simulink model "PubIfDecisionTOS_MDL"  (R2020b)
settings: configuration reference "DspaceConfig" (kept outside this file)
PostLoadFcn:
  | if any(exist('dsrtsu_mdlpostloadfcn', 'file') ~= 0), dsrtsu_mdlpostloadfcn('Execute', bdroot); end
InitFcn:
  | , if any(exist('dsmpb_private', 'file') ~= 0), dsmpb_private('dsmpb_mdlclblib', 'Init', bdroot); end,
undefined symbols (not defined in the file or in its folder): C_TOS_ACCEgoRAxletoFbumplength_m, C_TOS_ACCTargetFront_Flag, C_TOS_AEBJAPedObjDxThre_Val, C_TOS_AEBJAPedObjDyThre_Val, C_TOS_AEBJATargetSize_Val, C_TOS_AEBJAVehObjDxThre_Val, C_TOS_AEBJAVehObjDyThre_Val, C_TOS_AEBJuncPedTargetSize_Val, C_TOS_AEBLatObjDxThre_Val, C_TOS_AEBLatPedDyThre_Val, C_TOS_AEBLatTargetSize_Val, C_TOS_AEBLongTargetInEgoFront_Flag, C_TOS_axAbsGround_Parameter, C_TOS_CameraConfirmedFlag, C_TOS_CNsubjWidth, C_TOS_CurrentLaneCoreMinWidth_Val, C_TOS_CutInProb_Val_Zero, C_TOS_CutOutProb_Val_Zero, C_TOS_D2R_Val, C_TOS_DefaultValueObjectToCenterLine_dy, C_TOS_EgoCarWidth_Val, C_TOS_EgoDxRefPoint_m, C_TOS_EgoRAxletoFbumplength_m, C_TOS_HalfWidthVehicle_Con, C_TOS_HWA_CurrentLaneFlag, C_TOS_HWA_LeftLaneFlag, C_TOS_HWA_MovingDir_Vaild, C_TOS_HWA_MovState_Vaild, C_TOS_HWA_RightLaneFlag, C_TOS_LaneLineCourseErrorFront, C_TOS_LaneLineCourseErrorRear, C_TOS_MotorbikeDefaultWidth_m, C_TOS_NumberOfEffectiveTargets, C_TOS_Obj_Age_Val, C_TOS_Objdx_Constraint_Val, C_TOS_ObjectDefaultWidth_m, C_TOS_ObjInCurrentLane_Val, C_TOS_ObjInCurrentLaneValid, C_TOS_ObjInLeftLaneValid, C_TOS_ObjInRightLaneValid, C_TOS_ObjNotInCurrentLane_Val, C_TOS_ObjNotREElementType, C_TOS_ObjPredictDis_dy_ConstantVal_Zeros, C_TOS_ObjToCenterLine_ConstantVal_Zeros, C_TOS_OFMObjIDInvilad_Val, C_TOS_PIL_LatDisCons_Val_zero, C_TOS_PIL_ObjectCutInFlag_b, C_TOS_PIL_ObjectCutOutFlag_b, C_TOS_PIL_ObjLaneProb_al_Val, C_TOS_PP_ObjFusType_FC_Confirm_b, C_TOS_PP_ObjFusType_FC_FR_Confirm_b, C_TOS_PP_ObjFusType_FR_Confirm_b, C_TOS_RE_80BoolDefault_Val, C_TOS_RE_80Single181Default_Val, C_TOS_RE_80Single255Default_Val, C_TOS_RE_80Uint8Default_Val, C_TOS_RE_D2R, C_TOS_RE_D_180_Val, C_TOS_RE_InvalidObjectID_Val, C_TOS_RE_InvalidTargetChainDir_Val ... (+142)
libraries: simulink x1650, TOS_LIB x361, canfdmsglib x14
(part 52 of 69)

== system PubIfDecisionTOS_MDL/TOS_20201112/TOS_2012080320/TOS/ACC/TOS_ACCRightLane/ACC_LeftLane_Target/TOS_ACC_P3/ACC_P3_Targe/ACC_P3_Targe/TOS_ACC_ObjTypeConfirm/Subsystem1 ==
  note: 针对有选中的运动目标，运动状态突变为静止，改变其运动状态为运动
  object_MovingState : Inport
  ACC_Target_ID_K1 : Inport  Port=2
  ACC_Target_ID_K2 : Inport  Port=3
  ACC_Target_MovState_K1 : Inport  Port=4
  ACC_Target_MovState_K2 : Inport  Port=5
  ObjectID : Inport  Port=6
  Object_Type : Inport  Port=7
  Compare To Constant11 : simulink/Logic and Bit Operations/Compare To Constant  relop===  const=1  OutDataTypeStr=boolean
  Compare To Constant2 : simulink/Logic and Bit Operations/Compare To Constant  relop===  const=OFM_OBJ_MOVINGSTATE_E.MOVING  OutDataTypeStr=boolean
      settings: AttributesFormatString=OFM_OBJ_MOVINGSTATE_E.MOVING = 2
  Compare To Constant3 : simulink/Logic and Bit Operations/Compare To Constant  relop===  const=OFM_OBJ_MOVINGSTATE_E.MOVING_SLOWLY  OutDataTypeStr=boolean
      settings: AttributesFormatString=OFM_OBJ_MOVINGSTATE_E.MOVING_SLOWLY = 5
  Compare To Constant6 : simulink/Logic and Bit Operations/Compare To Constant  relop===  const=OFM_OBJ_MOVINGSTATE_E.STOPPED  OutDataTypeStr=boolean
      settings: AttributesFormatString=OFM_OBJ_MOVINGSTATE_E.STOPPED = 4
  Compare To Constant8 : simulink/Logic and Bit Operations/Compare To Constant  relop===  const=OFM_OBJ_TYPE_E.UNKNOWN_TYPE  OutDataTypeStr=boolean
      settings: AttributesFormatString=OFM_OBJ_TYPE_E.UNKNOWN_TYPE = 1
  Data Type Conversion2 : DataTypeConversion  OutDataTypeStr=Enum: OFM_OBJ_MOVINGSTATE_E
  Logical Operator : Logic  AllPortsSameDT=off  OutDataTypeStr=boolean
  Logical Operator2 : Logic  Operator=OR  Inputs=4  AllPortsSameDT=off  OutDataTypeStr=boolean
  Subsystem : Subsystem
  Output : Outport
  wires:
  ACC_Target_MovState_K2/1 -> Subsystem/5(ACC_Target_MovState_K2)
  Subsystem/1(TOS_ObjMovStateCfm) -> Compare To Constant11/1
  Data Type Conversion2/1 -> Compare To Constant2/1, Compare To Constant3/1, Compare To Constant6/1, Subsystem/1(ObjMovState)
  ObjectID/1 -> [ObjectID], Subsystem/6(ObjectID)
  ACC_Target_ID_K1/1 -> Subsystem/2(ACC_Target_ID_K1), [ACC_Target_ID_K1]
  Compare To Constant11/1 -> Logical Operator2/4
  Logical Operator2/1 -> Logical Operator/1
  ACC_Target_MovState_K1/1 -> Subsystem/4(ACC_Target_MovState_K1)
  Compare To Constant2/1 -> Logical Operator2/1
  Compare To Constant3/1 -> Logical Operator2/2
  Compare To Constant8/1 -> Logical Operator/2
  ACC_Target_ID_K2/1 -> Subsystem/3(ACC_Target_ID_K2)
  object_MovingState/1 -> Data Type Conversion2/1
  Compare To Constant6/1 -> Logical Operator2/3
  Object_Type/1 -> Compare To Constant8/1
  Logical Operator/1 -> Output/1

== system PubIfDecisionTOS_MDL/TOS_20201112/TOS_2012080320/TOS/ACC/TOS_ACCRightLane/ACC_LeftLane_Target/TOS_ACC_P3/ACC_P3_Targe/ACC_P3_Targe/TOS_ACC_ObjTypeConfirm/TOS_ACCObjTypeAborDly ==
  ACC_Target_ID_K1 : Inport
  ObjectID : Inport  Port=2
  TOS_ACCObjType : Inport  Port=3
  If : If  IfExpression=u1
  If Action Subsystem : Subsystem  TreatAsAtomicUnit=on
  If Action Subsystem1 : Subsystem  TreatAsAtomicUnit=on
  Merge : Merge
  Relational Operator : RelationalOperator  Operator===  OutDataTypeStr=boolean  RndMeth=Simplest
  TOS_ACCObjTypeFilt : Outport
  wires:
  Merge/1 -> TOS_ACCObjTypeFilt/1
  If Action Subsystem/1(TOS_ACCFusionTypeFilt) -> Merge/2
  If Action Subsystem1/1(TOS_ACCFusionTypeFilt) -> Merge/1
  Relational Operator/1 -> If/1
  ObjectID/1 -> Relational Operator/2
  ACC_Target_ID_K1/1 -> Relational Operator/1
  If/2 -> If Action Subsystem/Action
  TOS_ACCObjType/1 -> If Action Subsystem/1(TOS_ACCFusionType), If Action Subsystem1/1(TOS_ACCFusionType)
  If/1 -> If Action Subsystem1/Action

== system PubIfDecisionTOS_MDL/TOS_20201112/TOS_2012080320/TOS/ACC/TOS_ACCRightLane/ACC_LeftLane_Target/TOS_ACC_P3/ACC_P3_Targe/ACC_P3_Targe/TOS_ACC_ObstacleProbConfirm/TOS_ACCObstacleProbAborDly ==
  ACC_Target_ID_K1 : Inport
  ObjectID : Inport  Port=2
  TOS_ACCObstacleProb : Inport  Port=3
  If : If  IfExpression=u1
  If Action Subsystem : Subsystem  TreatAsAtomicUnit=on
  If Action Subsystem1 : Subsystem  TreatAsAtomicUnit=on
  Merge : Merge
  Subsystem : Subsystem
  TOS_ACCObstacleProbFilt : Outport
  wires:
  Merge/1 -> TOS_ACCObstacleProbFilt/1
  If Action Subsystem/1(TOS_ACCFusionTypeFilt) -> Merge/2
  If Action Subsystem1/1(TOS_ACCFusionTypeFilt) -> Merge/1
  Subsystem/1(ACC_SameTargetP0) -> If/1
  ObjectID/1 -> Subsystem/2(ObjectID)
  ACC_Target_ID_K1/1 -> Subsystem/1(ACC_TargetP0_ID_K1)
  If/2 -> If Action Subsystem/Action
  TOS_ACCObstacleProb/1 -> If Action Subsystem/1(TOS_ACCFusionType), If Action Subsystem1/1(TOS_ACCFusionType)
  If/1 -> If Action Subsystem1/Action

== system PubIfDecisionTOS_MDL/TOS_20201112/TOS_2012080320/TOS/ACC/TOS_ACCRightLane/ACC_LeftLane_Target/TOS_ACC_P3/ACC_P3_Targe/ACC_P3_Targe/TOS_ACC_TargetMovingDirConfirm/Subsystem ==
  ObjMovState : Inport
  ACC_Target_ID_K1 : Inport  Port=2
  ACC_Target_ID_K2 : Inport  Port=3
  ACC_Target_MovState_K1 : Inport  Port=4
  ACC_Target_MovState_K2 : Inport  Port=5
  ObjectID : Inport  Port=6
  TOS_ObjMovStateCfmFlow : Stateflow chart  TreatAsAtomicUnit=on
  TOS_ObjMovStateCfm : Outport
  wires:
  ObjectID/1 -> TOS_ObjMovStateCfmFlow/6(ObjectID)
  ObjMovState/1 -> TOS_ObjMovStateCfmFlow/5(ObjMovState)
  ACC_Target_MovState_K2/1 -> TOS_ObjMovStateCfmFlow/4(Target_MovState_K2)
  ACC_Target_MovState_K1/1 -> TOS_ObjMovStateCfmFlow/3(Target_MovState_K1)
  ACC_Target_ID_K2/1 -> TOS_ObjMovStateCfmFlow/2(Target_ID_K2)
  ACC_Target_ID_K1/1 -> TOS_ObjMovStateCfmFlow/1(Target_ID_K1)
  TOS_ObjMovStateCfmFlow/1(TOS_ObjMovStateCfm) -> TOS_ObjMovStateCfm/1

== system PubIfDecisionTOS_MDL/TOS_20201112/TOS_2012080320/TOS/ACC/TOS_ACCRightLane/ACC_LeftLane_Target/TOS_ACC_P3/ACC_P3_Targe/ACC_P3_Targe/TOS_ACC_TargetMovingDirConfirm/TOS_ACCMovingDirAborDly ==
  ACC_TargetP0_ID_K1 : Inport
  ObjectID : Inport  Port=2
  TOS_ACCMovingDir : Inport  Port=3
  If : If  IfExpression=u1
  If Action Subsystem : Subsystem  TreatAsAtomicUnit=on
  If Action Subsystem1 : Subsystem  TreatAsAtomicUnit=on
  Merge : Merge
  Subsystem : Subsystem
  TOS_ACC_TrgMovDirFlag_6_ObserVale : Outport
  TOS_ACC_TrgMovDir : Outport  Port=2
  wires:
  Merge/1 -> TOS_ACC_TrgMovDir/1
  If Action Subsystem/1(TOS_ACCMovingDirFilt) -> Merge/2
  If Action Subsystem1/1(TOS_ACCMovingDirFilt) -> Merge/1
  Subsystem/1(ACC_SameTargetP0) -> If/1, TOS_ACC_TrgMovDirFlag_6_ObserVale/1
  ObjectID/1 -> Subsystem/2(ObjectID)
  ACC_TargetP0_ID_K1/1 -> Subsystem/1(ACC_TargetP0_ID_K1)
  If/2 -> If Action Subsystem/Action
  TOS_ACCMovingDir/1 -> If Action Subsystem/1(TOS_ACCMovingDir), If Action Subsystem1/1(TOS_ACCMovingDir)
  If/1 -> If Action Subsystem1/Action

== system PubIfDecisionTOS_MDL/TOS_20201112/TOS_2012080320/TOS/ACC/TOS_ACCRightLane/ACC_LeftLane_Target/TOS_ACC_P5/ACC_P5_Targe/ACC_P5_Targe/TOS_ACC_FusionTypeConfirm/Subsystem1 ==
  ObjMovState : Inport
  ACC_Target_ID_K1 : Inport  Port=2
  ACC_Target_ID_K2 : Inport  Port=3
  ACC_Target_MovState_K1 : Inport  Port=4
  ACC_Target_MovState_K2 : Inport  Port=5
  ObjectID : Inport  Port=6
  TOS_ObjMovStateCfmFlow1 : Stateflow chart  TreatAsAtomicUnit=on
  TOS_ObjMovStateCfm : Outport
  wires:
  TOS_ObjMovStateCfmFlow1/1(TOS_ObjMovStateCfm) -> TOS_ObjMovStateCfm/1
  ACC_Target_ID_K1/1 -> TOS_ObjMovStateCfmFlow1/1(Target_ID_K1)
  ACC_Target_ID_K2/1 -> TOS_ObjMovStateCfmFlow1/2(Target_ID_K2)
  ACC_Target_MovState_K1/1 -> TOS_ObjMovStateCfmFlow1/3(Target_MovState_K1)
  ACC_Target_MovState_K2/1 -> TOS_ObjMovStateCfmFlow1/4(Target_MovState_K2)
  ObjMovState/1 -> TOS_ObjMovStateCfmFlow1/5(ObjMovState)
  ObjectID/1 -> TOS_ObjMovStateCfmFlow1/6(ObjectID)

== system PubIfDecisionTOS_MDL/TOS_20201112/TOS_2012080320/TOS/ACC/TOS_ACCRightLane/ACC_LeftLane_Target/TOS_ACC_P5/ACC_P5_Targe/ACC_P5_Targe/TOS_ACC_FusionTypeConfirm/TOS_ACCFusionTypeAborDly ==
  ACC_TargetP0_ID_K1 : Inport
  ObjectID : Inport  Port=2
  TOS_ACCFusionType : Inport  Port=3
  If : If  IfExpression=u1
  If Action Subsystem : Subsystem  TreatAsAtomicUnit=on
  If Action Subsystem1 : Subsystem  TreatAsAtomicUnit=on
  Merge : Merge
  Relational Operator : RelationalOperator  Operator===  OutDataTypeStr=boolean  RndMeth=Simplest
  TOS_ACCFusionTypeFilt : Outport
  wires:
  If/1 -> If Action Subsystem1/Action
  TOS_ACCFusionType/1 -> If Action Subsystem1/1(TOS_ACCFusionType), If Action Subsystem/1(TOS_ACCFusionType)
  If/2 -> If Action Subsystem/Action
  ACC_TargetP0_ID_K1/1 -> Relational Operator/1
  ObjectID/1 -> Relational Operator/2
  Relational Operator/1 -> If/1
  If Action Subsystem1/1(TOS_ACCFusionTypeFilt) -> Merge/1
  If Action Subsystem/1(TOS_ACCFusionTypeFilt) -> Merge/2
  Merge/1 -> TOS_ACCFusionTypeFilt/1

== system PubIfDecisionTOS_MDL/TOS_20201112/TOS_2012080320/TOS/ACC/TOS_ACCRightLane/ACC_LeftLane_Target/TOS_ACC_P5/ACC_P5_Targe/ACC_P5_Targe/TOS_ACC_ObjTypeConfirm/Subsystem1 ==
  note: 针对有选中的运动目标，运动状态突变为静止，改变其运动状态为运动
  object_MovingState : Inport
  ACC_Target_ID_K1 : Inport  Port=2
  ACC_Target_ID_K2 : Inport  Port=3
  ACC_Target_MovState_K1 : Inport  Port=4
  ACC_Target_MovState_K2 : Inport  Port=5
  ObjectID : Inport  Port=6
  Object_Type : Inport  Port=7
  Compare To Constant11 : simulink/Logic and Bit Operations/Compare To Constant  relop===  const=1  OutDataTypeStr=boolean
  Compare To Constant2 : simulink/Logic and Bit Operations/Compare To Constant  relop===  const=OFM_OBJ_MOVINGSTATE_E.MOVING  OutDataTypeStr=boolean
      settings: AttributesFormatString=OFM_OBJ_MOVINGSTATE_E.MOVING = 2
  Compare To Constant3 : simulink/Logic and Bit Operations/Compare To Constant  relop===  const=OFM_OBJ_MOVINGSTATE_E.MOVING_SLOWLY  OutDataTypeStr=boolean
      settings: AttributesFormatString=OFM_OBJ_MOVINGSTATE_E.MOVING_SLOWLY = 5
  Compare To Constant6 : simulink/Logic and Bit Operations/Compare To Constant  relop===  const=OFM_OBJ_MOVINGSTATE_E.STOPPED  OutDataTypeStr=boolean
      settings: AttributesFormatString=OFM_OBJ_MOVINGSTATE_E.STOPPED = 4
  Compare To Constant8 : simulink/Logic and Bit Operations/Compare To Constant  relop===  const=OFM_OBJ_TYPE_E.UNKNOWN_TYPE  OutDataTypeStr=boolean
      settings: AttributesFormatString=OFM_OBJ_TYPE_E.UNKNOWN_TYPE = 1
  Data Type Conversion2 : DataTypeConversion  OutDataTypeStr=Enum: OFM_OBJ_MOVINGSTATE_E
  Logical Operator : Logic  AllPortsSameDT=off  OutDataTypeStr=boolean
  Logical Operator2 : Logic  Operator=OR  Inputs=4  AllPortsSameDT=off  OutDataTypeStr=boolean
  Subsystem : Subsystem
  Output : Outport
  wires:
  Logical Operator/1 -> Output/1
  Object_Type/1 -> Compare To Constant8/1
  Compare To Constant6/1 -> Logical Operator2/3
  object_MovingState/1 -> Data Type Conversion2/1
  ACC_Target_ID_K2/1 -> Subsystem/3(ACC_Target_ID_K2)
  Compare To Constant8/1 -> Logical Operator/2
  Compare To Constant3/1 -> Logical Operator2/2
  Compare To Constant2/1 -> Logical Operator2/1
  ACC_Target_MovState_K1/1 -> Subsystem/4(ACC_Target_MovState_K1)
  Logical Operator2/1 -> Logical Operator/1
  Compare To Constant11/1 -> Logical Operator2/4
  ACC_Target_ID_K1/1 -> [ACC_Target_ID_K1], Subsystem/2(ACC_Target_ID_K1)
  ObjectID/1 -> Subsystem/6(ObjectID), [ObjectID]
  Data Type Conversion2/1 -> Subsystem/1(ObjMovState), Compare To Constant6/1, Compare To Constant3/1, Compare To Constant2/1
  Subsystem/1(TOS_ObjMovStateCfm) -> Compare To Constant11/1
  ACC_Target_MovState_K2/1 -> Subsystem/5(ACC_Target_MovState_K2)

== system PubIfDecisionTOS_MDL/TOS_20201112/TOS_2012080320/TOS/ACC/TOS_ACCRightLane/ACC_LeftLane_Target/TOS_ACC_P5/ACC_P5_Targe/ACC_P5_Targe/TOS_ACC_ObjTypeConfirm/TOS_ACCObjTypeAborDly ==
  ACC_Target_ID_K1 : Inport
  ObjectID : Inport  Port=2
  TOS_ACCObjType : Inport  Port=3
  If : If  IfExpression=u1
  If Action Subsystem : Subsystem  TreatAsAtomicUnit=on
  If Action Subsystem1 : Subsystem  TreatAsAtomicUnit=on
  Merge : Merge
  Relational Operator : RelationalOperator  Operator===  OutDataTypeStr=boolean  RndMeth=Simplest
  TOS_ACCObjTypeFilt : Outport
  wires:
  If/1 -> If Action Subsystem1/Action
  TOS_ACCObjType/1 -> If Action Subsystem1/1(TOS_ACCFusionType), If Action Subsystem/1(TOS_ACCFusionType)
  If/2 -> If Action Subsystem/Action
  ACC_Target_ID_K1/1 -> Relational Operator/1
  ObjectID/1 -> Relational Operator/2
  Relational Operator/1 -> If/1
  If Action Subsystem1/1(TOS_ACCFusionTypeFilt) -> Merge/1
  If Action Subsystem/1(TOS_ACCFusionTypeFilt) -> Merge/2
  Merge/1 -> TOS_ACCObjTypeFilt/1

== system PubIfDecisionTOS_MDL/TOS_20201112/TOS_2012080320/TOS/ACC/TOS_ACCRightLane/ACC_LeftLane_Target/TOS_ACC_P5/ACC_P5_Targe/ACC_P5_Targe/TOS_ACC_ObstacleProbConfirm/TOS_ACCObstacleProbAborDly ==
  ACC_Target_ID_K1 : Inport
  ObjectID : Inport  Port=2
  TOS_ACCObstacleProb : Inport  Port=3
  If : If  IfExpression=u1
  If Action Subsystem : Subsystem  TreatAsAtomicUnit=on
  If Action Subsystem1 : Subsystem  TreatAsAtomicUnit=on
  Merge : Merge
  Subsystem : Subsystem
  TOS_ACCObstacleProbFilt : Outport
  wires:
  If/1 -> If Action Subsystem1/Action
  TOS_ACCObstacleProb/1 -> If Action Subsystem1/1(TOS_ACCFusionType), If Action Subsystem/1(TOS_ACCFusionType)
  If/2 -> If Action Subsystem/Action
  ACC_Target_ID_K1/1 -> Subsystem/1(ACC_TargetP0_ID_K1)
  ObjectID/1 -> Subsystem/2(ObjectID)
  Subsystem/1(ACC_SameTargetP0) -> If/1
  If Action Subsystem1/1(TOS_ACCFusionTypeFilt) -> Merge/1
  If Action Subsystem/1(TOS_ACCFusionTypeFilt) -> Merge/2
  Merge/1 -> TOS_ACCObstacleProbFilt/1

== system PubIfDecisionTOS_MDL/TOS_20201112/TOS_2012080320/TOS/ACC/TOS_ACCRightLane/ACC_LeftLane_Target/TOS_ACC_P5/ACC_P5_Targe/ACC_P5_Targe/TOS_ACC_TargetMovingDirConfirm/Subsystem ==
  ObjMovState : Inport
  ACC_Target_ID_K1 : Inport  Port=2
  ACC_Target_ID_K2 : Inport  Port=3
  ACC_Target_MovState_K1 : Inport  Port=4
  ACC_Target_MovState_K2 : Inport  Port=5
  ObjectID : Inport  Port=6
  TOS_ObjMovStateCfmFlow : Stateflow chart  TreatAsAtomicUnit=on
  TOS_ObjMovStateCfm : Outport
  wires:
  TOS_ObjMovStateCfmFlow/1(TOS_ObjMovStateCfm) -> TOS_ObjMovStateCfm/1
  ACC_Target_ID_K1/1 -> TOS_ObjMovStateCfmFlow/1(Target_ID_K1)
  ACC_Target_ID_K2/1 -> TOS_ObjMovStateCfmFlow/2(Target_ID_K2)
  ACC_Target_MovState_K1/1 -> TOS_ObjMovStateCfmFlow/3(Target_MovState_K1)
  ACC_Target_MovState_K2/1 -> TOS_ObjMovStateCfmFlow/4(Target_MovState_K2)
  ObjMovState/1 -> TOS_ObjMovStateCfmFlow/5(ObjMovState)
  ObjectID/1 -> TOS_ObjMovStateCfmFlow/6(ObjectID)

== system PubIfDecisionTOS_MDL/TOS_20201112/TOS_2012080320/TOS/ACC/TOS_ACCRightLane/ACC_LeftLane_Target/TOS_ACC_P5/ACC_P5_Targe/ACC_P5_Targe/TOS_ACC_TargetMovingDirConfirm/TOS_ACCMovingDirAborDly ==
  ACC_TargetP0_ID_K1 : Inport
  ObjectID : Inport  Port=2
  TOS_ACCMovingDir : Inport  Port=3
  If : If  IfExpression=u1
  If Action Subsystem : Subsystem  TreatAsAtomicUnit=on
  If Action Subsystem1 : Subsystem  TreatAsAtomicUnit=on
  Merge : Merge
  Subsystem : Subsystem
  TOS_ACC_TrgMovDirFlag_6_ObserVale : Outport
  TOS_ACC_TrgMovDir : Outport  Port=2
  wires:
  If/1 -> If Action Subsystem1/Action
  TOS_ACCMovingDir/1 -> If Action Subsystem1/1(TOS_ACCMovingDir), If Action Subsystem/1(TOS_ACCMovingDir)
  If/2 -> If Action Subsystem/Action
  ACC_TargetP0_ID_K1/1 -> Subsystem/1(ACC_TargetP0_ID_K1)
  ObjectID/1 -> Subsystem/2(ObjectID)
  Subsystem/1(ACC_SameTargetP0) -> TOS_ACC_TrgMovDirFlag_6_ObserVale/1, If/1
  If Action Subsystem1/1(TOS_ACCMovingDirFilt) -> Merge/1
  If Action Subsystem/1(TOS_ACCMovingDirFilt) -> Merge/2
  Merge/1 -> TOS_ACC_TrgMovDir/1

== system PubIfDecisionTOS_MDL/TOS_20201112/TOS_2012080320/TOS/AEB/TOS_AEBJunct1105/AEBJunc_Object_Condition/AEBJA_TargetCondition/TOS_AEBJunc_TargetsCondition/AEBJunc_PedTargetCondition/AEBJunc_PedTargetMoveDir/TOS_AEBJuncTargetCrossing ==
  Object_Infor : Inport
  Abs : Abs
  Abs1 : Abs
  Abs2 : Abs
  Add : Sum
  Bus Selector : BusSelector  OutputSignals=PP_ObjMovingDirSignalProcessing,Object_HeadingAngle
  Bus Selector1 : BusSelector  OutputSignals=Object_VY
  Bus Selector2 : BusSelector  OutputSignals=Object_VX,VIE_EgoVelocity
  Bus Selector3 : BusSelector  OutputSignals=Object_Dy
  Compare To Constant : simulink/Logic and Bit Operations/Compare To Constant  relop=<  const=P_TOS_CrossingTarget_VxabsOffset_val  OutDataTypeStr=boolean
      settings: AttributesFormatString=%<const>
  Compare To Constant1 : simulink/Logic and Bit Operations/Compare To Constant  relop=>  const=P_TOS_CrossingTargetVyvThre_val  OutDataTypeStr=boolean
      settings: AttributesFormatString=%<const>
  Compare To Constant15 : simulink/Logic and Bit Operations/Compare To Constant  relop=>=  const=P_TOS_ObjLatCroYawAngMinThre_Val  OutDataTypeStr=boolean
      settings: AttributesFormatString=P_TOS_ObjLatCroYawAngMinThre_Val = 45
  Compare To Constant16 : simulink/Logic and Bit Operations/Compare To Constant  relop=<=  const=P_TOS_ObjLatCroYawAngMaxThre_Val  OutDataTypeStr=boolean
      settings: AttributesFormatString=P_TOS_ObjLatCroYawAngMaxThre_Val = 135
  Compare To Constant2 : simulink/Logic and Bit Operations/Compare To Constant  relop===  const=ObjectMovingOrientation_E.Crossing  OutDataTypeStr=boolean
      settings: AttributesFormatString=%<const>
  Data Type Conversion2 : DataTypeConversion  OutDataTypeStr=Enum: ObjectMovingOrientation_E
  Demux : Demux  Outputs=3
  Demux1 : Demux  Outputs=3
  Logical Operator : Logic  Operator=OR  Inputs=3  AllPortsSameDT=off  OutDataTypeStr=boolean
  Logical Operator{1..4,10} (5 alike) : Logic  AllPortsSameDT=off  OutDataTypeStr=boolean
  Logical Operator5 : Logic  Operator=OR  AllPortsSameDT=off  OutDataTypeStr=boolean
  Relational Operator : RelationalOperator  Operator=<  OutDataTypeStr=boolean  RndMeth=Simplest
  Relational Operator1 : RelationalOperator  Operator=<  OutDataTypeStr=boolean  RndMeth=Simplest
  Relational Operator2 : RelationalOperator  Operator=>  OutDataTypeStr=boolean  RndMeth=Simplest
  Relational Operator3 : RelationalOperator  Operator=>  OutDataTypeStr=boolean  RndMeth=Simplest
  Tapped Delay : simulink/Discrete/Tapped Delay  vinit=0.0  samptime=-1  NumDelays=2  DelayOrder=Oldest  includeCurrent=on
  TOS_AEBJuncTargetCrossingFlg : Outport
  wires:
  Bus Selector/2 -> Abs/1  "<Object_HeadingAngle>"
  Logical Operator/1 -> TOS_AEBJuncTargetCrossingFlg/1
  Demux/2 -> Relational Operator3/1, Relational Operator2/2
  Demux1/3 -> Relational Operator1/2
  Relational Operator2/1 -> Logical Operator3/1
  Compare To Constant2/1 -> Logical Operator/1
  Bus Selector2/1 -> Add/1  "<Object_VX>"
  Logical Operator1/1 -> Logical Operator2/1
  Demux/1 -> Relational Operator2/1
  Compare To Constant16/1 -> Logical Operator10/2
  Compare To Constant15/1 -> Logical Operator10/1
  Logical Operator10/1 -> Logical Operator/2
  Add/1 -> Abs1/1
  Compare To Constant1/1 -> Logical Operator1/2
  Abs/1 -> Compare To Constant16/1, Compare To Constant15/1
  Relational Operator3/1 -> Logical Operator3/2
  Logical Operator4/1 -> Logical Operator5/2
  Bus Selector3/1 -> Tapped Delay/1  "<Object_Dy>"
  Data Type Conversion2/1 -> Compare To Constant2/1
  Relational Operator1/1 -> Logical Operator4/2
  Logical Operator3/1 -> Logical Operator5/1
  Logical Operator5/1 -> Logical Operator2/2
  Demux1/2 -> Relational Operator1/1, Relational Operator/2
  Abs1/1 -> Compare To Constant/1
  Compare To Constant/1 -> Logical Operator1/1
  Tapped Delay/1 -> Demux1/1, Demux/1
  Bus Selector/1 -> Data Type Conversion2/1  "<PP_ObjMovingDirSignalProcessing>"
  Demux1/1 -> Relational Operator/1
  Object_Infor/1 -> Bus Selector2/1, Bus Selector1/1, Bus Selector3/1, Bus Selector/1
  Relational Operator/1 -> Logical Operator4/1
  Abs2/1 -> Compare To Constant1/1
  Bus Selector1/1 -> Abs2/1  "<Object_VY>"
  Logical Operator2/1 -> Logical Operator/3
  Demux/3 -> Relational Operator3/2
  Bus Selector2/2 -> Add/2  "<VIE_EgoVelocity>"

== system PubIfDecisionTOS_MDL/TOS_20201112/TOS_2012080320/TOS/AEB/TOS_AEBJunct1105/AEBJunc_Object_Condition/AEBJA_TargetCondition/TOS_AEBJunc_TargetsCondition/AEBJunc_PedTargetCondition/AEBJunc_PedTargetMoveDir/TOS_AEBJuncTargetOncoming ==
  Object_Infor : Inport
  Abs{,1..3} (4 alike) : Abs
  Add{,2..4} (4 alike) : Sum
  Add1 : Sum  Inputs=+-
  Bus Selector : BusSelector  OutputSignals=PP_ObjMovingDirSignalProcessing,Object_HeadingAngle
  Bus Selector1 : BusSelector  OutputSignals=VIE_EgoVelocity
  Bus Selector2 : BusSelector  OutputSignals=Object_VX,VIE_EgoVelocity,Object_VY
  Bus Selector3 : BusSelector  OutputSignals=axvRefMs2
  Bus Selector4 : BusSelector  OutputSignals=Object_Dx
  Compare To Constant : simulink/Logic and Bit Operations/Compare To Constant  relop=<  const=P_TOS_OncomingTarget_VxabsOffset_val  OutDataTypeStr=boolean
      settings: AttributesFormatString=%<const> = -0.7m/s
  Compare To Constant1 : simulink/Logic and Bit Operations/Compare To Constant  relop=>  const=P_TOS_CrossingTargetVyvThre_val  OutDataTypeStr=boolean
      settings: AttributesFormatString=%<const>
  Compare To Constant16 : simulink/Logic and Bit Operations/Compare To Constant  relop=>  const=P_TOS_ObjLatCroYawAngMaxThre_Val  OutDataTypeStr=boolean
      settings: AttributesFormatString=P_TOS_ObjLatCroYawAngMaxThre_Val = 135
  Compare To Constant2 : simulink/Logic and Bit Operations/Compare To Constant  relop===  const=ObjectMovingOrientation_E.OnComingDir  OutDataTypeStr=boolean
      settings: AttributesFormatString=%<const>
  Compare To Constant3 : simulink/Logic and Bit Operations/Compare To Constant  relop=>  const=P_TOS_ObjOncomingYawAngMaxThre_Val  OutDataTypeStr=boolean
      settings: AttributesFormatString=P_TOS_ObjOncomingYawAngMaxThre_Val = 180
  Compare To Constant4 : simulink/Logic and Bit Operations/Compare To Constant  relop=<  const=0  OutDataTypeStr=boolean
  Constant : Constant  Value=C_TOS_StepTime_Val
  Constant1 : Constant  Value=C_TOS_StepTime_Val
  Constant2 : Constant  Value=P_TOS_OncomingPedDxChangeOffset_Val
  Data Type Conversion2 : DataTypeConversion  OutDataTypeStr=Enum: ObjectMovingOrientation_E
  Gain : Gain  Gain=1/2
  Gain1 : Gain  Gain=1/2
  Logical Operator : Logic  Operator=OR  Inputs=4  AllPortsSameDT=off  OutDataTypeStr=boolean
  Logical Operator{1..3,10} (4 alike) : Logic  AllPortsSameDT=off  OutDataTypeStr=boolean
  Math Function : Math  Operator=square  SaturateOnIntegerOverflow=on
  Product : Product
  Product1 : Product
  Relational Operator : RelationalOperator  Operator=>  OutDataTypeStr=boolean  RndMeth=Simplest
  Unit Delay{,1..3} (4 alike) : UnitDelay  InitialCondition=255  SampleTime=-1  HasFrameUpgradeWarning=on
  TOS_AEBJuncTargetOncomingFlg : Outport
  wires:
  Bus Selector2/2 -> Add/2  "<VIE_EgoVelocity>"
  Logical Operator1/1 -> Logical Operator/3
  Abs2/1 -> Compare To Constant1/1
  Object_Infor/1 -> Bus Selector/1, Bus Selector3/1, Bus Selector1/1, Bus Selector4/1, Bus Selector2/1
  Bus Selector/1 -> Data Type Conversion2/1  "<PP_ObjMovingDirSignalProcessing>"
  Compare To Constant/1 -> Logical Operator1/1
  Abs1/1 -> Compare To Constant/1
  Data Type Conversion2/1 -> Compare To Constant2/1
  Abs/1 -> Compare To Constant3/1, Compare To Constant16/1
  Compare To Constant1/1 -> Logical Operator1/2
  Add/1 -> Abs1/1
  Logical Operator10/1 -> Logical Operator/2
  Compare To Constant16/1 -> Logical Operator10/1
  Bus Selector2/1 -> Add/1  "<Object_VX>"
  Compare To Constant2/1 -> Logical Operator/1
  Logical Operator/1 -> TOS_AEBJuncTargetOncomingFlg/1
  Bus Selector/2 -> Abs/1  "<Object_HeadingAngle>"
  Compare To Constant3/1 -> Logical Operator10/2
  Bus Selector4/1 -> Unit Delay/1, Add1/1  "<Object_Dx>"
  Unit Delay/1 -> Add1/2
  Add1/1 -> Abs3/1, Compare To Constant4/1
  Compare To Constant4/1 -> Logical Operator2/1
  Bus Selector2/3 -> Abs2/1  "<Object_VY>"
  Abs3/1 -> Relational Operator/1
  Bus Selector1/1 -> Unit Delay2/1  "<VIE_EgoVelocity>"
  Constant/1 -> Product/2
  Constant1/1 -> Math Function/1
  Math Function/1 -> Product1/2
  Product1/1 -> Gain/1
  Gain/1 -> Add2/2
  Product/1 -> Add2/1
  Bus Selector3/1 -> Unit Delay1/1, Add3/1  "<axvRefMs2>"
  Add2/1 -> Add4/1
  Relational Operator/1 -> Logical Operator3/1, Unit Delay3/1
  Logical Operator2/1 -> Logical Operator/4
  Unit Delay1/1 -> Add3/2
  Add3/1 -> Gain1/1
  Gain1/1 -> Product1/1
  Unit Delay2/1 -> Product/1
  Constant2/1 -> Add4/2
  Add4/1 -> Relational Operator/2
  Unit Delay3/1 -> Logical Operator3/2
  Logical Operator3/1 -> Logical Operator2/2

== system PubIfDecisionTOS_MDL/TOS_20201112/TOS_2012080320/TOS/AEB/TOS_AEBJunct1105/AEBJunc_Object_Condition/AEBJA_TargetCondition/TOS_AEBJunc_TargetsCondition/AEBJunc_PedTargetCondition/AEBJunc_PedTargetObjectTypeFlag/AEBJunc_PedTargetObjectTypeAborDly ==
  AEBJunc_PedTarget_ID_K1 : Inport
  ObjectID : Inport  Port=2
  TOS_AEBJunc_PedObjectType : Inport  Port=3
  Compare To Constant : simulink/Logic and Bit Operations/Compare To Constant  relop=>=  const=1  OutDataTypeStr=boolean
  If : If  IfExpression=u1
  If Action Subsystem : Subsystem  TreatAsAtomicUnit=on
  If Action Subsystem1 : Subsystem  TreatAsAtomicUnit=on
  Merge : Merge
  Subsystem : Subsystem
  Sum of Elements : Sum  Inputs=+
  TOS_AEBJunc_PedObjectTypeFilt : Outport
  wires:
  If/1 -> If Action Subsystem1/Action
  TOS_AEBJunc_PedObjectType/1 -> If Action Subsystem1/1(TOS_AEBJunc_PedObjectType), If Action Subsystem/1(TOS_AEBJunc_PedObjectType)
  If/2 -> If Action Subsystem/Action
  AEBJunc_PedTarget_ID_K1/1 -> Subsystem/1(AEBJunc_PedTarget_ID_K1)
  ObjectID/1 -> Subsystem/2(ObjectID)
  Subsystem/1(AEBJunc_PedSameTarget) -> Sum of Elements/1
  If Action Subsystem1/1(TOS_AEBJunc_PedObjectTypeFilt) -> Merge/1
  If Action Subsystem/1(TOS_AEBJunc_PedObjectTypeFilt) -> Merge/2
  Merge/1 -> TOS_AEBJunc_PedObjectTypeFilt/1
  Sum of Elements/1 -> Compare To Constant/1
  Compare To Constant/1 -> If/1

== system PubIfDecisionTOS_MDL/TOS_20201112/TOS_2012080320/TOS/AEB/TOS_AEBJunct1105/AEBJunc_Object_Condition/AEBJA_TargetCondition/TOS_AEBJunc_TargetsCondition/AEBJunc_VehTargetCondition/AEBJunc_VehTargetObjectTypeFlag/AEBJunc_VehTargetObjectTypeAborDly ==
  AEBJunc_VehTarget_ID_K1 : Inport
  ObjectID : Inport  Port=2
  TOS_AEBJunc_VehObjectType : Inport  Port=3
  Compare To Constant : simulink/Logic and Bit Operations/Compare To Constant  relop=>=  const=1  OutDataTypeStr=boolean
  If : If  IfExpression=u1
  If Action Subsystem : Subsystem  TreatAsAtomicUnit=on
  If Action Subsystem1 : Subsystem  TreatAsAtomicUnit=on
  Merge : Merge
  Subsystem : Subsystem
  Sum of Elements : Sum  Inputs=+
  TOS_AEBJunc_VehObjectTypeFilt : Outport
  wires:
  If/1 -> If Action Subsystem1/Action
  TOS_AEBJunc_VehObjectType/1 -> If Action Subsystem1/1(TOS_AEBJunc_VehObjectType), If Action Subsystem/1(TOS_AEBJunc_VehObjectType)
  If/2 -> If Action Subsystem/Action
  AEBJunc_VehTarget_ID_K1/1 -> Subsystem/1(AEBJunc_VehTarget_ID_K1)
  ObjectID/1 -> Subsystem/2(ObjectID)
  Subsystem/1(AEBJunc_VehSameTarget) -> Sum of Elements/1
  If Action Subsystem1/1(TOS_AEBJunc_VehObjectTypeFilt) -> Merge/1
  If Action Subsystem/1(TOS_AEBJJunc_VehObjectTypeFilt) -> Merge/2
  Merge/1 -> TOS_AEBJunc_VehObjectTypeFilt/1
  Sum of Elements/1 -> Compare To Constant/1
  Compare To Constant/1 -> If/1

== system PubIfDecisionTOS_MDL/TOS_20201112/TOS_2012080320/TOS/AEB/TOS_AEBJunct1105/AEBJunc_Object_Condition1/AEBJA_TargetCondition/TOS_AEBJunc_TargetsCondition/AEBJunc_PedTargetCondition/AEBJunc_PedTargetMoveDir/TOS_AEBJuncTargetCrossing ==
  Object_Infor : Inport
  Abs : Abs
  Abs1 : Abs
  Abs2 : Abs
  Add : Sum
  Bus Selector : BusSelector  OutputSignals=PP_ObjMovingDirSignalProcessing,Object_HeadingAngle
  Bus Selector1 : BusSelector  OutputSignals=Object_VY
  Bus Selector2 : BusSelector  OutputSignals=Object_VX,VIE_EgoVelocity
  Bus Selector3 : BusSelector  OutputSignals=Object_Dy
  Compare To Constant : simulink/Logic and Bit Operations/Compare To Constant  relop=<  const=P_TOS_CrossingTarget_VxabsOffset_val  OutDataTypeStr=boolean
      settings: AttributesFormatString=%<const>
  Compare To Constant1 : simulink/Logic and Bit Operations/Compare To Constant  relop=>  const=P_TOS_CrossingTargetVyvThre_val  OutDataTypeStr=boolean
      settings: AttributesFormatString=%<const>
  Compare To Constant15 : simulink/Logic and Bit Operations/Compare To Constant  relop=>=  const=P_TOS_ObjLatCroYawAngMinThre_Val  OutDataTypeStr=boolean
      settings: AttributesFormatString=P_TOS_ObjLatCroYawAngMinThre_Val = 45
  Compare To Constant16 : simulink/Logic and Bit Operations/Compare To Constant  relop=<=  const=P_TOS_ObjLatCroYawAngMaxThre_Val  OutDataTypeStr=boolean
      settings: AttributesFormatString=P_TOS_ObjLatCroYawAngMaxThre_Val = 135
  Compare To Constant2 : simulink/Logic and Bit Operations/Compare To Constant  relop===  const=ObjectMovingOrientation_E.Crossing  OutDataTypeStr=boolean
      settings: AttributesFormatString=%<const>
  Data Type Conversion2 : DataTypeConversion  OutDataTypeStr=Enum: ObjectMovingOrientation_E
  Demux : Demux  Outputs=3
  Demux1 : Demux  Outputs=3
  Logical Operator : Logic  Operator=OR  Inputs=3  AllPortsSameDT=off  OutDataTypeStr=boolean
  Logical Operator{1..4,10} (5 alike) : Logic  AllPortsSameDT=off  OutDataTypeStr=boolean
  Logical Operator5 : Logic  Operator=OR  AllPortsSameDT=off  OutDataTypeStr=boolean
  Relational Operator : RelationalOperator  Operator=<  OutDataTypeStr=boolean  RndMeth=Simplest
  Relational Operator1 : RelationalOperator  Operator=<  OutDataTypeStr=boolean  RndMeth=Simplest
  Relational Operator2 : RelationalOperator  Operator=>  OutDataTypeStr=boolean  RndMeth=Simplest
  Relational Operator3 : RelationalOperator  Operator=>  OutDataTypeStr=boolean  RndMeth=Simplest
  Tapped Delay : simulink/Discrete/Tapped Delay  vinit=0.0  samptime=-1  NumDelays=2  DelayOrder=Oldest  includeCurrent=on
  TOS_AEBJuncTargetCrossingFlg : Outport
  wires:
  Bus Selector2/2 -> Add/2  "<VIE_EgoVelocity>"
  Demux/3 -> Relational Operator3/2
  Logical Operator2/1 -> Logical Operator/3
  Bus Selector1/1 -> Abs2/1  "<Object_VY>"
  Abs2/1 -> Compare To Constant1/1
  Relational Operator/1 -> Logical Operator4/1
  Object_Infor/1 -> Bus Selector/1, Bus Selector3/1, Bus Selector1/1, Bus Selector2/1
  Demux1/1 -> Relational Operator/1
  Bus Selector/1 -> Data Type Conversion2/1  "<PP_ObjMovingDirSignalProcessing>"
  Tapped Delay/1 -> Demux/1, Demux1/1
  Compare To Constant/1 -> Logical Operator1/1
  Abs1/1 -> Compare To Constant/1
  Demux1/2 -> Relational Operator/2, Relational Operator1/1
  Logical Operator5/1 -> Logical Operator2/2
  Logical Operator3/1 -> Logical Operator5/1
  Relational Operator1/1 -> Logical Operator4/2
  Data Type Conversion2/1 -> Compare To Constant2/1
  Bus Selector3/1 -> Tapped Delay/1  "<Object_Dy>"
  Logical Operator4/1 -> Logical Operator5/2
  Relational Operator3/1 -> Logical Operator3/2
  Abs/1 -> Compare To Constant15/1, Compare To Constant16/1
  Compare To Constant1/1 -> Logical Operator1/2
  Add/1 -> Abs1/1
  Logical Operator10/1 -> Logical Operator/2
  Compare To Constant15/1 -> Logical Operator10/1
  Compare To Constant16/1 -> Logical Operator10/2
  Demux/1 -> Relational Operator2/1
  Logical Operator1/1 -> Logical Operator2/1
  Bus Selector2/1 -> Add/1  "<Object_VX>"
  Compare To Constant2/1 -> Logical Operator/1
  Relational Operator2/1 -> Logical Operator3/1
  Demux1/3 -> Relational Operator1/2
  Demux/2 -> Relational Operator2/2, Relational Operator3/1
  Logical Operator/1 -> TOS_AEBJuncTargetCrossingFlg/1
  Bus Selector/2 -> Abs/1  "<Object_HeadingAngle>"

== system PubIfDecisionTOS_MDL/TOS_20201112/TOS_2012080320/TOS/AEB/TOS_AEBJunct1105/AEBJunc_Object_Condition1/AEBJA_TargetCondition/TOS_AEBJunc_TargetsCondition/AEBJunc_PedTargetCondition/AEBJunc_PedTargetMoveDir/TOS_AEBJuncTargetOncoming ==
  Object_Infor : Inport
  Abs{,1..3} (4 alike) : Abs
  Add{,2..4} (4 alike) : Sum
  Add1 : Sum  Inputs=+-
  Bus Selector : BusSelector  OutputSignals=PP_ObjMovingDirSignalProcessing,Object_HeadingAngle
  Bus Selector1 : BusSelector  OutputSignals=VIE_EgoVelocity
  Bus Selector2 : BusSelector  OutputSignals=Object_VX,VIE_EgoVelocity,Object_VY
  Bus Selector3 : BusSelector  OutputSignals=axvRefMs2
  Bus Selector4 : BusSelector  OutputSignals=Object_Dx
  Compare To Constant : simulink/Logic and Bit Operations/Compare To Constant  relop=<  const=P_TOS_OncomingTarget_VxabsOffset_val  OutDataTypeStr=boolean
      settings: AttributesFormatString=%<const> = -0.7m/s
  Compare To Constant1 : simulink/Logic and Bit Operations/Compare To Constant  relop=>  const=P_TOS_CrossingTargetVyvThre_val  OutDataTypeStr=boolean
      settings: AttributesFormatString=%<const>
  Compare To Constant16 : simulink/Logic and Bit Operations/Compare To Constant  relop=>  const=P_TOS_ObjLatCroYawAngMaxThre_Val  OutDataTypeStr=boolean
      settings: AttributesFormatString=P_TOS_ObjLatCroYawAngMaxThre_Val = 135
  Compare To Constant2 : simulink/Logic and Bit Operations/Compare To Constant  relop===  const=ObjectMovingOrientation_E.OnComingDir  OutDataTypeStr=boolean
      settings: AttributesFormatString=%<const>
  Compare To Constant3 : simulink/Logic and Bit Operations/Compare To Constant  relop=>  const=P_TOS_ObjOncomingYawAngMaxThre_Val  OutDataTypeStr=boolean
      settings: AttributesFormatString=P_TOS_ObjOncomingYawAngMaxThre_Val = 180
  Compare To Constant4 : simulink/Logic and Bit Operations/Compare To Constant  relop=<  const=0  OutDataTypeStr=boolean
  Constant : Constant  Value=C_TOS_StepTime_Val
  Constant1 : Constant  Value=C_TOS_StepTime_Val
  Constant2 : Constant  Value=P_TOS_OncomingPedDxChangeOffset_Val
  Data Type Conversion2 : DataTypeConversion  OutDataTypeStr=Enum: ObjectMovingOrientation_E
  Gain : Gain  Gain=1/2
  Gain1 : Gain  Gain=1/2
  Logical Operator : Logic  Operator=OR  Inputs=4  AllPortsSameDT=off  OutDataTypeStr=boolean
  Logical Operator{1..3,10} (4 alike) : Logic  AllPortsSameDT=off  OutDataTypeStr=boolean
  Math Function : Math  Operator=square  SaturateOnIntegerOverflow=on
  Product : Product
  Product1 : Product
  Relational Operator : RelationalOperator  Operator=>  OutDataTypeStr=boolean  RndMeth=Simplest
  Unit Delay{,1..3} (4 alike) : UnitDelay  InitialCondition=255  SampleTime=-1  HasFrameUpgradeWarning=on
  TOS_AEBJuncTargetOncomingFlg : Outport
  wires:
  Logical Operator3/1 -> Logical Operator2/2
  Unit Delay3/1 -> Logical Operator3/2
  Add4/1 -> Relational Operator/2
  Constant2/1 -> Add4/2
  Unit Delay2/1 -> Product/1
  Gain1/1 -> Product1/1
  Add3/1 -> Gain1/1
  Unit Delay1/1 -> Add3/2
  Logical Operator2/1 -> Logical Operator/4
  Relational Operator/1 -> Unit Delay3/1, Logical Operator3/1
  Add2/1 -> Add4/1
  Bus Selector3/1 -> Add3/1, Unit Delay1/1  "<axvRefMs2>"
  Product/1 -> Add2/1
  Gain/1 -> Add2/2
  Product1/1 -> Gain/1
  Math Function/1 -> Product1/2
  Constant1/1 -> Math Function/1
  Constant/1 -> Product/2
  Bus Selector1/1 -> Unit Delay2/1  "<VIE_EgoVelocity>"
  Abs3/1 -> Relational Operator/1
  Bus Selector2/3 -> Abs2/1  "<Object_VY>"
  Compare To Constant4/1 -> Logical Operator2/1
  Add1/1 -> Compare To Constant4/1, Abs3/1
  Unit Delay/1 -> Add1/2
  Bus Selector4/1 -> Add1/1, Unit Delay/1  "<Object_Dx>"
  Compare To Constant3/1 -> Logical Operator10/2
  Bus Selector/2 -> Abs/1  "<Object_HeadingAngle>"
  Logical Operator/1 -> TOS_AEBJuncTargetOncomingFlg/1
  Compare To Constant2/1 -> Logical Operator/1
  Bus Selector2/1 -> Add/1  "<Object_VX>"
  Compare To Constant16/1 -> Logical Operator10/1
  Logical Operator10/1 -> Logical Operator/2
  Add/1 -> Abs1/1
  Compare To Constant1/1 -> Logical Operator1/2
  Abs/1 -> Compare To Constant16/1, Compare To Constant3/1
  Data Type Conversion2/1 -> Compare To Constant2/1
  Abs1/1 -> Compare To Constant/1
  Compare To Constant/1 -> Logical Operator1/1
  Bus Selector/1 -> Data Type Conversion2/1  "<PP_ObjMovingDirSignalProcessing>"
  Object_Infor/1 -> Bus Selector2/1, Bus Selector4/1, Bus Selector1/1, Bus Selector3/1, Bus Selector/1
  Abs2/1 -> Compare To Constant1/1
  Logical Operator1/1 -> Logical Operator/3
  Bus Selector2/2 -> Add/2  "<VIE_EgoVelocity>"

== system PubIfDecisionTOS_MDL/TOS_20201112/TOS_2012080320/TOS/AEB/TOS_AEBJunct1105/AEBJunc_Object_Condition1/AEBJA_TargetCondition/TOS_AEBJunc_TargetsCondition/AEBJunc_PedTargetCondition/AEBJunc_PedTargetObjectTypeFlag/AEBJunc_PedTargetObjectTypeAborDly ==
  AEBJunc_PedTarget_ID_K1 : Inport
  ObjectID : Inport  Port=2
  TOS_AEBJunc_PedObjectType : Inport  Port=3
  Compare To Constant : simulink/Logic and Bit Operations/Compare To Constant  relop=>=  const=1  OutDataTypeStr=boolean
  If : If  IfExpression=u1
  If Action Subsystem : Subsystem  TreatAsAtomicUnit=on
  If Action Subsystem1 : Subsystem  TreatAsAtomicUnit=on
  Merge : Merge
  Subsystem : Subsystem
  Sum of Elements : Sum  Inputs=+
  TOS_AEBJunc_PedObjectTypeFilt : Outport
  wires:
  Compare To Constant/1 -> If/1
  Sum of Elements/1 -> Compare To Constant/1
  Merge/1 -> TOS_AEBJunc_PedObjectTypeFilt/1
  If Action Subsystem/1(TOS_AEBJunc_PedObjectTypeFilt) -> Merge/2
  If Action Subsystem1/1(TOS_AEBJunc_PedObjectTypeFilt) -> Merge/1
  Subsystem/1(AEBJunc_PedSameTarget) -> Sum of Elements/1
  ObjectID/1 -> Subsystem/2(ObjectID)
  AEBJunc_PedTarget_ID_K1/1 -> Subsystem/1(AEBJunc_PedTarget_ID_K1)
  If/2 -> If Action Subsystem/Action
  TOS_AEBJunc_PedObjectType/1 -> If Action Subsystem/1(TOS_AEBJunc_PedObjectType), If Action Subsystem1/1(TOS_AEBJunc_PedObjectType)
  If/1 -> If Action Subsystem1/Action

== system PubIfDecisionTOS_MDL/TOS_20201112/TOS_2012080320/TOS/AEB/TOS_AEBJunct1105/AEBJunc_Object_Condition1/AEBJA_TargetCondition/TOS_AEBJunc_TargetsCondition/AEBJunc_VehTargetCondition/AEBJunc_VehTargetObjectTypeFlag/AEBJunc_VehTargetObjectTypeAborDly ==
  AEBJunc_VehTarget_ID_K1 : Inport
  ObjectID : Inport  Port=2
  TOS_AEBJunc_VehObjectType : Inport  Port=3
  Compare To Constant : simulink/Logic and Bit Operations/Compare To Constant  relop=>=  const=1  OutDataTypeStr=boolean
  If : If  IfExpression=u1
  If Action Subsystem : Subsystem  TreatAsAtomicUnit=on
  If Action Subsystem1 : Subsystem  TreatAsAtomicUnit=on
  Merge : Merge
  Subsystem : Subsystem
  Sum of Elements : Sum  Inputs=+
  TOS_AEBJunc_VehObjectTypeFilt : Outport
  wires:
  Compare To Constant/1 -> If/1
  Sum of Elements/1 -> Compare To Constant/1
  Merge/1 -> TOS_AEBJunc_VehObjectTypeFilt/1
  If Action Subsystem/1(TOS_AEBJJunc_VehObjectTypeFilt) -> Merge/2
  If Action Subsystem1/1(TOS_AEBJunc_VehObjectTypeFilt) -> Merge/1
  Subsystem/1(AEBJunc_VehSameTarget) -> Sum of Elements/1
  ObjectID/1 -> Subsystem/2(ObjectID)
  AEBJunc_VehTarget_ID_K1/1 -> Subsystem/1(AEBJunc_VehTarget_ID_K1)
  If/2 -> If Action Subsystem/Action
  TOS_AEBJunc_VehObjectType/1 -> If Action Subsystem/1(TOS_AEBJunc_VehObjectType), If Action Subsystem1/1(TOS_AEBJunc_VehObjectType)
  If/1 -> If Action Subsystem1/Action

== system PubIfDecisionTOS_MDL/TOS_20201112/TOS_2012080320/TOS/AEB/TOS_AEBJunct_20201208/AEBJunc_Object_Condition/AEBJA_TargetCondition/TOS_AEBJunc_TargetsCondition/AEBJunc_PedTargetCondition/AEBJunc_PedTargetMoveDir/AEBLat_TargetMovDirAborDly ==
  AEBJunc_Target_ID_K1 : Inport
  ObjectID : Inport  Port=2
  TOS_AEBJunc_MovDir_Flag : Inport  Port=3
  Compare To Constant : simulink/Logic and Bit Operations/Compare To Constant  relop=>=  const=1  OutDataTypeStr=boolean
  If : If  IfExpression=u1
  If Action Subsystem : Subsystem  TreatAsAtomicUnit=on
  If Action Subsystem1 : Subsystem  TreatAsAtomicUnit=on
  Merge : Merge
  Subsystem : Subsystem
  Sum of Elements : Sum  Inputs=+
  TOS_AEBJunc_MovDirFlag_Delay : Outport
  wires:
  If/1 -> If Action Subsystem1/Action
  TOS_AEBJunc_MovDir_Flag/1 -> If Action Subsystem1/1(TOS_AEBJunc_MovDir_Flag), If Action Subsystem/1(TOS_AEBJunc_MovDir_Flag)
  If/2 -> If Action Subsystem/Action
  AEBJunc_Target_ID_K1/1 -> Subsystem/1(AEBJunc_Target_ID_K1)
  ObjectID/1 -> Subsystem/2(ObjectID)
  Subsystem/1(AEBJunc_SameTarget) -> Sum of Elements/1
  If Action Subsystem1/1(TOS_AEBJunc_MovDirFlag_Delay) -> Merge/1
  If Action Subsystem/1(TOS_AEBJunc_MovDirFlag) -> Merge/2
  Merge/1 -> TOS_AEBJunc_MovDirFlag_Delay/1
  Sum of Elements/1 -> Compare To Constant/1
  Compare To Constant/1 -> If/1

== system PubIfDecisionTOS_MDL/TOS_20201112/TOS_2012080320/TOS/AEB/TOS_AEBJunct_20201208/AEBJunc_Object_Condition/AEBJA_TargetCondition/TOS_AEBJunc_TargetsCondition/AEBJunc_PedTargetCondition/AEBJunc_PedTargetMoveDir/TOS_AEBJuncTargetCrossing ==
  Object_Infor : Inport
  Abs : Abs
  Abs1 : Abs
  Abs2 : Abs
  Add : Sum
  Bus Selector : BusSelector  OutputSignals=PP_ObjMovingDirSignalProcessing,Object_HeadingAngle
  Bus Selector1 : BusSelector  OutputSignals=Object_VY
  Bus Selector2 : BusSelector  OutputSignals=Object_VX,VIE_EgoVelocity
  Bus Selector3 : BusSelector  OutputSignals=Object_Dy
  Compare To Constant : simulink/Logic and Bit Operations/Compare To Constant  relop=<  const=P_TOS_CrossingTarget_VxabsOffset_val  OutDataTypeStr=boolean
      settings: AttributesFormatString=%<const>
  Compare To Constant1 : simulink/Logic and Bit Operations/Compare To Constant  relop=>  const=P_TOS_CrossingTargetVyvThre_val  OutDataTypeStr=boolean
      settings: AttributesFormatString=%<const>
  Compare To Constant15 : simulink/Logic and Bit Operations/Compare To Constant  relop=>=  const=P_TOS_ObjLatCroYawAngMinThre_Val  OutDataTypeStr=boolean
      settings: AttributesFormatString=P_TOS_ObjLatCroYawAngMinThre_Val = 45
  Compare To Constant16 : simulink/Logic and Bit Operations/Compare To Constant  relop=<=  const=P_TOS_ObjLatCroYawAngMaxThre_Val  OutDataTypeStr=boolean
      settings: AttributesFormatString=P_TOS_ObjLatCroYawAngMaxThre_Val = 135
  Compare To Constant2 : simulink/Logic and Bit Operations/Compare To Constant  relop===  const=ObjectMovingOrientation_E.Crossing  OutDataTypeStr=boolean
      settings: AttributesFormatString=%<const>
  Data Type Conversion2 : DataTypeConversion  OutDataTypeStr=Enum: ObjectMovingOrientation_E
  Demux : Demux  Outputs=3
  Demux1 : Demux  Outputs=3
  Logical Operator : Logic  Operator=OR  Inputs=3  AllPortsSameDT=off  OutDataTypeStr=boolean
  Logical Operator{1..4,10} (5 alike) : Logic  AllPortsSameDT=off  OutDataTypeStr=boolean
  Logical Operator5 : Logic  Operator=OR  AllPortsSameDT=off  OutDataTypeStr=boolean
  Relational Operator : RelationalOperator  Operator=<  OutDataTypeStr=boolean  RndMeth=Simplest
  Relational Operator1 : RelationalOperator  Operator=<  OutDataTypeStr=boolean  RndMeth=Simplest
  Relational Operator2 : RelationalOperator  Operator=>  OutDataTypeStr=boolean  RndMeth=Simplest
  Relational Operator3 : RelationalOperator  Operator=>  OutDataTypeStr=boolean  RndMeth=Simplest
  Tapped Delay : simulink/Discrete/Tapped Delay  vinit=0.0  samptime=-1  NumDelays=2  DelayOrder=Oldest  includeCurrent=on
  TOS_AEBJuncTargetCrossingFlg : Outport
  wires:
  Bus Selector/2 -> Abs/1  "<Object_HeadingAngle>"
  Logical Operator/1 -> TOS_AEBJuncTargetCrossingFlg/1
  Demux/2 -> Relational Operator3/1, Relational Operator2/2
  Demux1/3 -> Relational Operator1/2
  Relational Operator2/1 -> Logical Operator3/1
  Compare To Constant2/1 -> Logical Operator/1
  Bus Selector2/1 -> Add/1  "<Object_VX>"
  Logical Operator1/1 -> Logical Operator2/1
  Demux/1 -> Relational Operator2/1
  Compare To Constant16/1 -> Logical Operator10/2
  Compare To Constant15/1 -> Logical Operator10/1
  Logical Operator10/1 -> Logical Operator/2
  Add/1 -> Abs1/1
  Compare To Constant1/1 -> Logical Operator1/2
  Abs/1 -> Compare To Constant16/1, Compare To Constant15/1
  Relational Operator3/1 -> Logical Operator3/2
  Logical Operator4/1 -> Logical Operator5/2
  Bus Selector3/1 -> Tapped Delay/1  "<Object_Dy>"
  Data Type Conversion2/1 -> Compare To Constant2/1
  Relational Operator1/1 -> Logical Operator4/2
  Logical Operator3/1 -> Logical Operator5/1
  Logical Operator5/1 -> Logical Operator2/2
  Demux1/2 -> Relational Operator1/1, Relational Operator/2
  Abs1/1 -> Compare To Constant/1
  Compare To Constant/1 -> Logical Operator1/1
  Tapped Delay/1 -> Demux1/1, Demux/1
  Bus Selector/1 -> Data Type Conversion2/1  "<PP_ObjMovingDirSignalProcessing>"
  Demux1/1 -> Relational Operator/1
  Object_Infor/1 -> Bus Selector2/1, Bus Selector1/1, Bus Selector3/1, Bus Selector/1
  Relational Operator/1 -> Logical Operator4/1
  Abs2/1 -> Compare To Constant1/1
  Bus Selector1/1 -> Abs2/1  "<Object_VY>"
  Logical Operator2/1 -> Logical Operator/3
  Demux/3 -> Relational Operator3/2
  Bus Selector2/2 -> Add/2  "<VIE_EgoVelocity>"
